simulink model "helicopter_sysID_sim_21b"  (R2021b)
settings: Solver=FixedStepAuto  StartTime=0.0  StopTime=100  FixedStep=0.001  RelTol=1e-3
values from neighbouring files (symbols this model uses):
  helicopterSysID_neg = greyest(helicopterSysData_neg,helicopterSysGrey_neg,opt_greyest)    [helicopter_sysID.m]
  helicopterSysID_pos = greyest(helicopterSysData_pos,helicopterSysGrey_pos,opt_greyest)    [helicopter_sysID.m]
undefined symbols (not defined in the file or in its folder): neg, pos
settings Model: Creator=slmnu  LastModifiedBy=slmnu
settings DataIOCC: ReturnWorkspaceOutputs=off
settings DebuggingCC: UnconnectedInputMsg=none  UnconnectedOutputMsg=none  UnconnectedLineMsg=none
settings ModelReferenceCC: EnableRefExpFcnMdlSchedulingChecks=off
settings RTWCC: GPUComputeCapability=5.0  DLArmComputeVersion=20.02.1

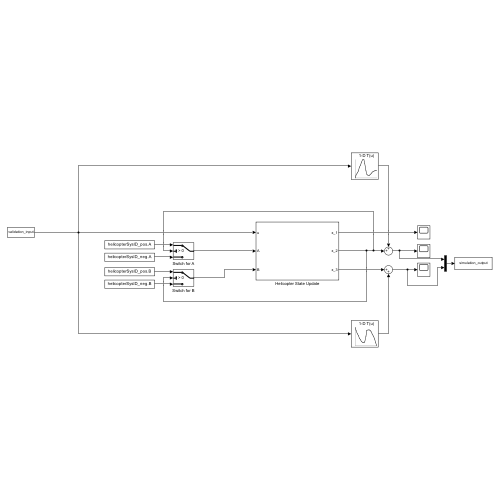
[thumbnail: Simulink's stored preview of the top-level diagram]
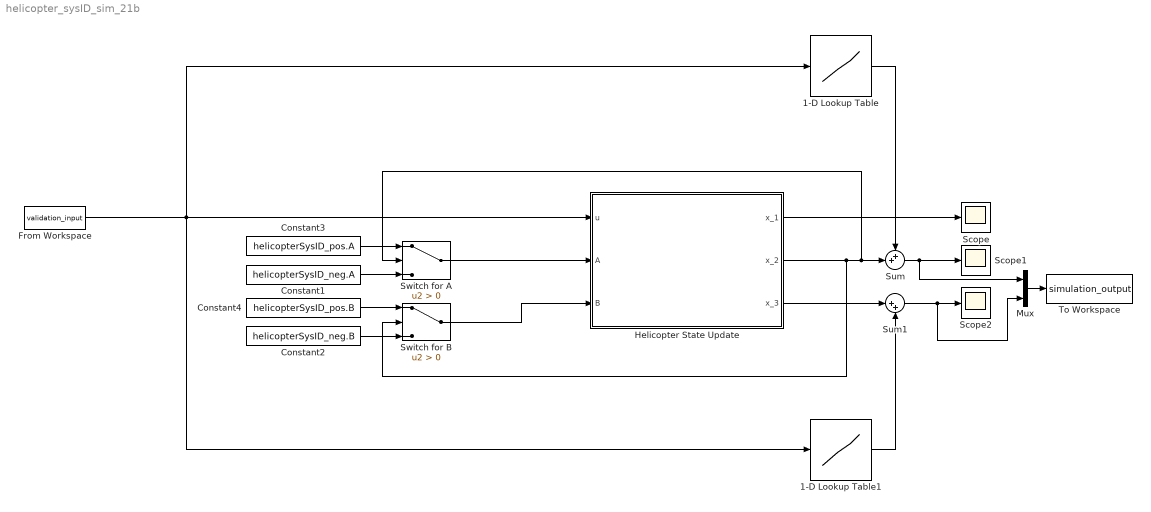
== system helicopter_sysID_sim_21b ==
  1-D Lookup Table : Lookup_n-D  NumberOfTableDimensions=1  BreakpointsForDimension1=-1:0.1:1  Table=[neg.pitch_offset 0 pos.pitch_offset]  InternalRulePriority=Speed  RndMeth=Simplest  InputSameDT=on
  1-D Lookup Table1 : Lookup_n-D  NumberOfTableDimensions=1  BreakpointsForDimension1=-1:0.1:1  Table=[neg.angular_velocity_offset 0 pos.angular_velocity_offset]  InternalRulePriority=Speed  RndMeth=Simplest  InputSameDT=on
  Constant1 : Constant  Value=helicopterSysID_neg.A
  Constant2 : Constant  Value=helicopterSysID_neg.B
  Constant3 : Constant  Value=helicopterSysID_pos.A
  Constant4 : Constant  Value=helicopterSysID_pos.B
  From Workspace : FromWorkspace  VariableName=validation_input
  Helicopter State Update : Subsystem
  Mux : Mux  Inputs=2
  Scope : Scope
  Scope1 : Scope
  Scope2 : Scope
  Sum : Sum  Inputs=++|
  Sum1 : Sum  Inputs=|++
  Switch for A : Switch  Criteria=u2 > Threshold
  Switch for B : Switch  Criteria=u2 > Threshold
  To Workspace : ToWorkspace  VariableName=simulation_output  SaveFormat=Timeseries  SampleTime=-1
  wires:
  Switch for A/1 -> Helicopter State Update/2(A)
  Constant1/1 -> Switch for A/3
  Constant2/1 -> Switch for B/3
  Constant4/1 -> Switch for B/1
  From Workspace/1 -> 1-D Lookup Table1/1, 1-D Lookup Table/1, Helicopter State Update/1(u)
  Constant3/1 -> Switch for A/1
  Helicopter State Update/1(x_1) -> Scope/1
  Helicopter State Update/2(x_2) -> Switch for B/2, Sum/2, Switch for A/2
  Switch for B/1 -> Helicopter State Update/3(B)
  Mux/1 -> To Workspace/1
  Sum/1 -> Mux/1, Scope1/1
  1-D Lookup Table/1 -> Sum/1
  Helicopter State Update/3(x_3) -> Sum1/1
  Sum1/1 -> Mux/2, Scope2/1
  1-D Lookup Table1/1 -> Sum1/2

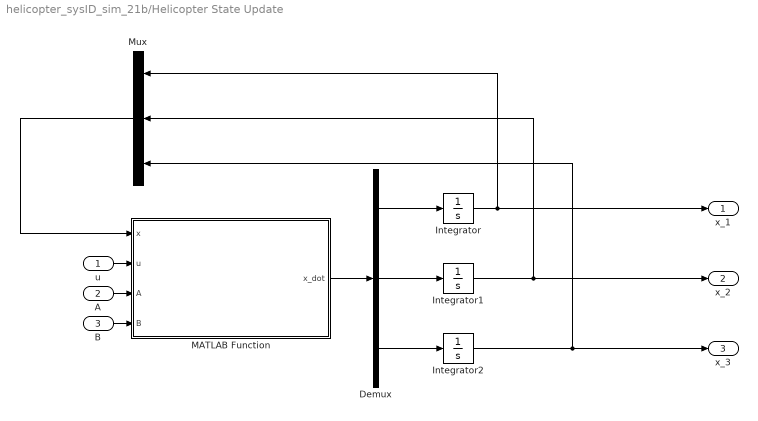
== system helicopter_sysID_sim_21b/Helicopter State Update ==
  u : Inport
  A : Inport  Port=2
  B : Inport  Port=3
  Demux : Demux  Outputs=3
  Integrator : Integrator
  Integrator1 : Integrator
  Integrator2 : Integrator
  MATLAB Function : MATLAB Function  TreatAsAtomicUnit=on
  Mux : Mux  Inputs=3
  x_1 : Outport
  x_2 : Outport  Port=2
  x_3 : Outport  Port=3
  wires:
  Demux/2 -> Integrator1/1
  Demux/1 -> Integrator/1
  Demux/3 -> Integrator2/1
  Mux/1 -> MATLAB Function/1(x)
  Integrator1/1 -> x_2/1, Mux/2
  Integrator2/1 -> x_3/1, Mux/3
  Integrator/1 -> x_1/1, Mux/1
  MATLAB Function/1(x_dot) -> Demux/1
  u/1 -> MATLAB Function/2(u)
  A/1 -> MATLAB Function/3(A)
  B/1 -> MATLAB Function/4(B)

== matlab function helicopter_sysID_sim_21b/Helicopter State Update/MATLAB Function ==
  data: x input; u input; x_dot output; A input; B input
function x_dot = state_update(x,u,A,B)

x_dot = A*x + B*u;
